simulink model "ulohaTri_simulink"  (R2022b)
settings: Solver=VariableStepAuto  StartTime=0.0  StopTime=10.0  RelTol=1e-3
model workspace (MAT data in the model file):
  a0 = -5
  a1 = -4
  a2 = 1
libraries: simulink x1
settings Model: Creator=marak  LastModifiedBy=marak

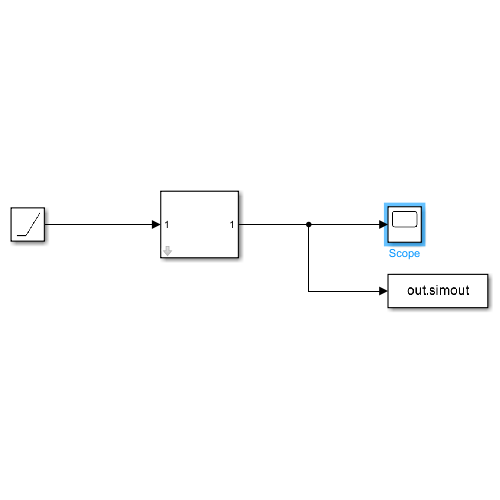
[thumbnail: Simulink's stored preview of the top-level diagram]
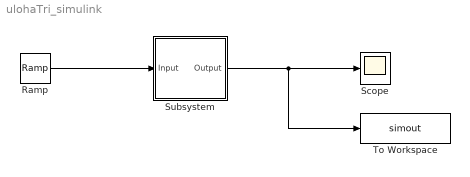
== system ulohaTri_simulink ==
  Ramp : simulink/Sources/Ramp  slope=1  start=0  InitialOutput=0
  Scope : Scope
  Subsystem : Subsystem  mask{a1=2, a2=2}
  To Workspace : ToWorkspace  VariableName=simout  SaveFormat=Timeseries  SampleTime=-1
  wires:
  Ramp/1 -> Subsystem/1(Input)
  Subsystem/1(Output) -> To Workspace/1, Scope/1

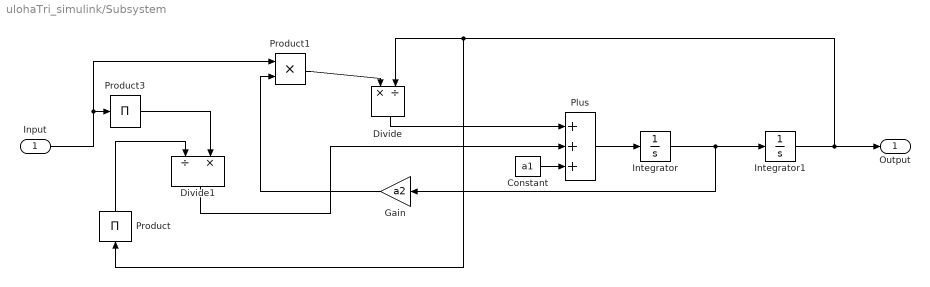
== system ulohaTri_simulink/Subsystem ==
  Input : Inport
  Constant : Constant  Value=a1
  Divide : Product  Inputs=*/  RndMeth=Zero  SaturateOnIntegerOverflow=on
  Divide1 : Product  Inputs=/*  RndMeth=Zero  SaturateOnIntegerOverflow=on
  Gain : Gain  Gain=a2
  Integrator : Integrator
  Integrator1 : Integrator  InitialCondition=1
  Plus : Sum  Inputs=+++
  Product : Product  Inputs=1
  Product1 : Product
  Product3 : Product  Inputs=1
  Output : Outport
  wires:
  Gain/1 -> Product1/2
  Integrator/1 -> Gain/1, Integrator1/1
  Constant/1 -> Plus/3
  Product1/1 -> Divide/1
  Divide1/1 -> Plus/2
  Integrator1/1 -> Product/1, Divide/2, Output/1
  Product3/1 -> Divide1/2
  Input/1 -> Product3/1, Product1/1
  Product/1 -> Divide1/1
  Divide/1 -> Plus/1
  Plus/1 -> Integrator/1
